simulink model "DirectnonLinearClosedLoop"  (Simulink 7.9)
settings: Solver=ode45  StartTime=0.0  StopTime=50  RelTol=1e-3
values from neighbouring files (symbols this model uses):
  K = lqr(A,B,Q,R)    [LQR.m]
settings Model: Creator=gdiazh  LastModifiedBy=root
settings OptimizationCC: InitFltsAndDblsToZero=on
settings DebuggingCC: FcnCallInpInsideContextMsg=Use local settings  StrictBusMsg=Warning
settings SFSimCC: SimParseCustomCode=off
settings GRTTargetCC: CombineOutputUpdateFcns=off  GRTInterface=on

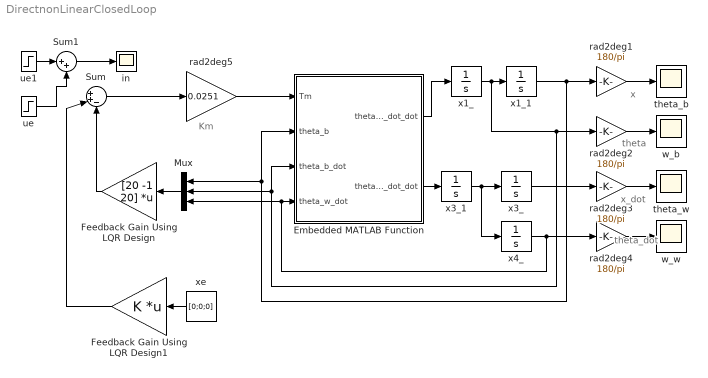
== system DirectnonLinearClosedLoop ==
  note: x
  note: x_dot
  note: theta_dot
  note: theta
  note: Km
  Embedded MATLAB Function : MATLAB Function  TreatAsAtomicUnit=on
  Feedback Gain Using LQR Design : Gain  Gain=[20 -1 20]  Multiplication=Matrix(K*u) (u vector)
  Feedback Gain Using LQR Design1 : Gain  Gain=K  Multiplication=Matrix(K*u) (u vector)
  Mux : Mux  Inputs=3
  Sum : Sum  Inputs=|++-
  Sum1 : Sum  Inputs=|++
  in : Scope
      settings: SaveName=position1
  rad2deg{1..4} (4 alike) : Gain  Gain=180/pi  SaturateOnIntegerOverflow=on  OutDataTypeStr=Inherit: Same as input  ParamDataTypeStr=Inherit: Same as input
  rad2deg5 : Gain  Gain=0.0251  SaturateOnIntegerOverflow=on  OutDataTypeStr=Inherit: Same as input  ParamDataTypeStr=Inherit: Same as input
  theta_b : Scope
      settings: SaveName=position
  theta_w : Scope
      settings: SaveName=linealVel
  ue : Step  After=0.1
  ue1 : Step  Time=2  After=-0.1
  w_b : Scope
      settings: TimeRange=0.35  YMin=88.25  YMax=91.75  SaveName=theta
  w_w : Scope
      settings: SaveName=angularVel
  x1_ : Integrator  UpperSaturationLimit=50  LowerSaturationLimit=-50
  x1_1 : Integrator  InitialCondition=-1  UpperSaturationLimit=50  LowerSaturationLimit=-50
  x3_ : Integrator  UpperSaturationLimit=100  LowerSaturationLimit=-100
  x3_1 : Integrator  UpperSaturationLimit=100  LowerSaturationLimit=-100
  x4_ : Integrator  UpperSaturationLimit=100  LowerSaturationLimit=-100
  xe : Constant  Value=[0;0;0]  VectorParams1D=off
  wires:
  rad2deg4/1 -> w_w/1
  rad2deg1/1 -> theta_b/1
  rad2deg3/1 -> theta_w/1
  x1_1/1 -> rad2deg1/1, Embedded MATLAB Function/2(theta_b), Mux/1
  x3_/1 -> rad2deg3/1
  x4_/1 -> rad2deg4/1, Embedded MATLAB Function/4(theta_w_dot), Mux/3
  rad2deg2/1 -> w_b/1
  Mux/1 -> Feedback Gain Using LQR Design/1
  xe/1 -> Feedback Gain Using LQR Design1/1
  Feedback Gain Using LQR Design/1 -> Sum/3
  x1_/1 -> x1_1/1, rad2deg2/1, Embedded MATLAB Function/3(theta_b_dot), Mux/2
  Embedded MATLAB Function/1(theta_b_dot_dot) -> x1_/1
  x3_1/1 -> x3_/1, x4_/1
  Embedded MATLAB Function/2(theta_w_dot_dot) -> x3_1/1
  Feedback Gain Using LQR Design1/1 -> Sum/2
  ue1/1 -> Sum1/1
  ue/1 -> Sum1/2
  Sum1/1 -> in/1
  rad2deg5/1 -> Embedded MATLAB Function/1(Tm)
  Sum/1 -> rad2deg5/1

== matlab function Embedded MATLAB Function ==
  data: Tm input double; theta_b input double; theta_b_dot input double; theta_w_dot input double; theta_b_dot_dot output double; theta_w_dot_dot output double
function [theta_b_dot_dot, theta_w_dot_dot] = nonLinearModel(Tm, theta_b, theta_b_dot, theta_w_dot)
    %Valores de los parametros
    
    l  = 7e-2;      %[m]
    lb = 6e-2;      %[m]
    mb = 222.2e-3;  %[Kg]
    mw = 22.9e-3;   %[Kg]
    Ib = 1.62e-3;   %[Kg m^2]
    Iw = 0.05e-3;   %[Kg m^2]
    Cb = 1.02e-3;   %[Kg m^2 s^-1]
    Cw = 0.05e-3;   %[Kg m^2 s^-1]
    g  = 9.8;       %[m/s^2]
    
    num1 = (mb*lb+mw*l)*g*sin(theta_b)-Tm-Cb*theta_b_dot+Cw*theta_w_dot;
    theta_b_dot_dot = num1/(Ib+mw*l^2);
    
    num2a = (Ib+Iw+mw*l^2)*(Tm-Cw*theta_w_dot);
    num2b = (mb*lb+mw*l)*g*sin(theta_b)-Cb*theta_b_dot;
    theta_w_dot_dot = num2a/(Iw*(Ib+mw*l^2))-num2b/(Ib+mw*l^2);
end

%Ib=(222÷6)×(12÷100)²+(222)×(7÷100)²
